simulink model "gpt_rdf1"  (R2013b)
settings: Solver=FixedStepDiscrete  StartTime=0.0  StopTime=4  FixedStep=1/800  RelTol=1e-3
libraries: commanapbnd3 x3
settings Model: Creator=rmg37  LastModifiedBy=rmg37
settings DataIOCC: SaveOutput=off  SaveTime=off
settings OptimizationCC: LocalBlockOutputs=off
settings DebuggingCC: AlgebraicLoopMsg=error  SingleTaskRateTransMsg=error

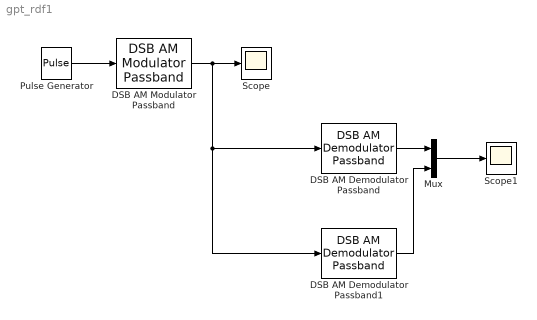
== system gpt_rdf1 ==
  DSB AM Demodulator Passband : commanapbnd3/DSB AM Demodulator Passband  Fc=99  Ph=0  method=Butterworth  n=4  cf=4  Rp=0.1  Rs=50  Offset=0
  DSB AM Demodulator Passband1 : commanapbnd3/DSB AM Demodulator Passband  Fc=99  Ph=pi/2  method=Butterworth  n=4  cf=4  Rp=0.1  Rs=50  Offset=0
  DSB AM Modulator Passband : commanapbnd3/DSB AM Modulator Passband  Fc=100  Ph=0  Offset=0
  Mux : Mux  Inputs=2
  Pulse Generator : DiscretePulseGenerator  PulseType=Time based  PulseWidth=50
  Scope : Scope
  Scope1 : Scope
  wires:
  Pulse Generator/1 -> DSB AM Modulator Passband/1
  DSB AM Modulator Passband/1 -> DSB AM Demodulator Passband1/1, DSB AM Demodulator Passband/1, Scope/1
  DSB AM Demodulator Passband/1 -> Mux/1
  Mux/1 -> Scope1/1
  DSB AM Demodulator Passband1/1 -> Mux/2
